simulink model "sliding_mode"  (R2025b)
settings: Solver=VariableStepAuto  StartTime=0.0  StopTime=50  RelTol=1e-3
libraries: simulink x2, slctrl_smc x1, matrix_library x1, cstblocks x1
settings Model: SimulationMode=rapid-accelerator  Creator=srivatsan  LastModifiedBy=srivatsan

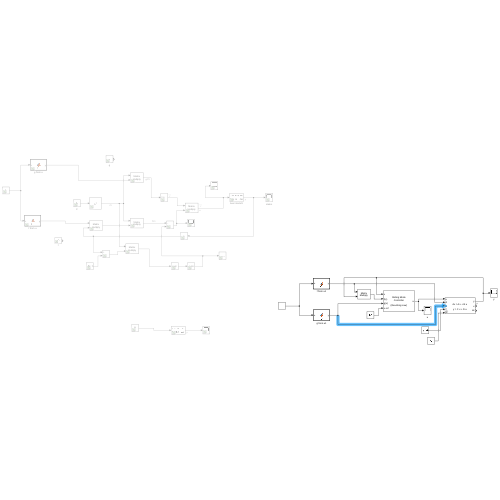
[thumbnail: Simulink's stored preview of the top-level diagram]
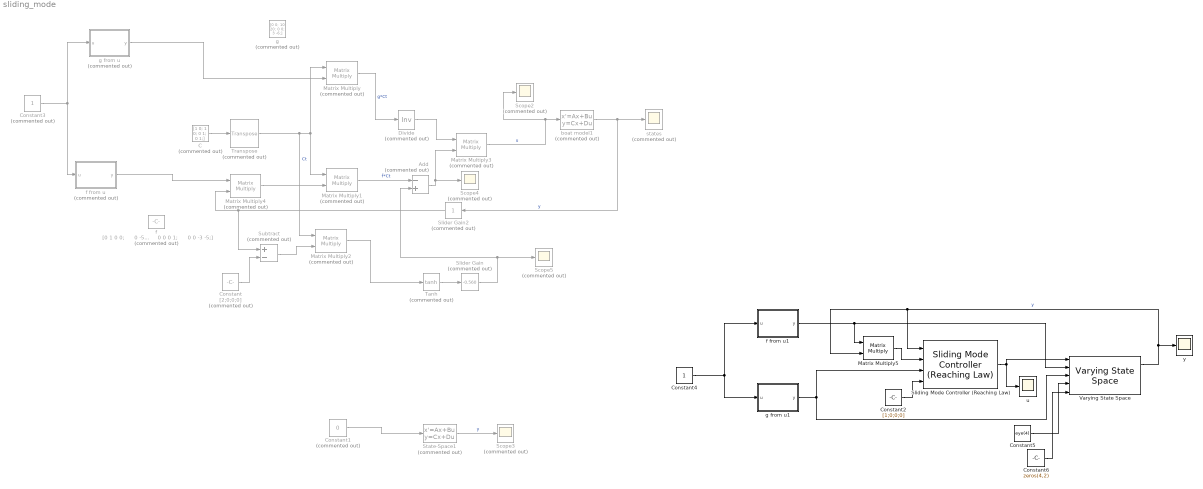
== system sliding_mode ==
  Add : Sum  Commented=on  Inputs=-+
  C : Constant  Commented=on  Value=[1 0; 1 0; 0 1; 0 1;]  VectorParams1D=off
  Constant : Constant  Commented=on  Value=[2;0;0;0]  VectorParams1D=off
  Constant1 : Constant  Commented=on  Value=0
  Constant2 : Constant  Value=[1;0;0;0]  VectorParams1D=off
  Constant3 : Constant  Commented=on
  Constant4 : Constant
  Constant5 : Constant  Value=eye(4)
  Constant6 : Constant  Value=zeros(4,2)
  Divide : Product  Commented=on  Inputs=/  Multiplication=Matrix(*)
  Matrix Multiply{,1..4} (5 alike) : Product  Commented=on  Multiplication=Matrix(*)
  Matrix Multiply5 : Product  Multiplication=Matrix(*)
  Scope{2..5} (4 alike) : Scope  Commented=on
      Scope2 settings: ActiveDisplayYMinimum=-0.20394139438387604  ActiveDisplayYMaximum=0.099478728460864418  DataLoggingVariableName=ScopeData2
      Scope3 settings: ActiveDisplayYMinimum=-7.1016769488332123  ActiveDisplayYMaximum=3.4136978035141685  DataLoggingVariableName=ScopeData3
      Scope4 settings: ActiveDisplayYMinimum=32.985672561237685  ActiveDisplayYMaximum=33.00453911435222  DataLoggingVariableName=ScopeData4
      Scope5 settings: ActiveDisplayYMinimum=-0.36552944112200225  ActiveDisplayYMaximum=0.6564815312712845  DataLoggingVariableName=ScopeData5
  Slider Gain : simulink/Math Operations/Slider Gain  Commented=on  gain=-0.560  low=-2  high=2
  Slider Gain2 : simulink/Math Operations/Slider Gain  Commented=on  gain=1  low=-2  high=2
  Sliding Mode Controller (Reaching Law) : slctrl_smc/Sliding Mode Controller (Reaching Law)  TaskMode=Tracking Mode  SlidingMatrix=[1 0;1 0;0 1;0 1]  EnableTrackingDerivative=off  EnableSwitchingFunction=off  ReachingLaw=Constant Rate  ReachingRate=1  ControlGain=0.01  PowerRate=0.01  BoundaryLayer=Hyperbolic Tangent  ZeroCross=off  Phi=0.01
  State-Space1 : StateSpace  Commented=on  A=[0,1;-10,-10]  B=[0;1;]  C=eye(2)  D=zeros(2,1)  InitialCondition=[5;3;]
  Subtract : Sum  Commented=on  Inputs=+-
  Tanh : Trigonometry  Commented=on  Operator=tanh
  Transpose : matrix_library/Transpose  Commented=on
  Varying State Space : cstblocks/Linear Parameter Varying/Varying State Space  InitialConditionSource=internal  InitialCondition=0  xNames=''  OutputX=on  OutputDX=on  Feedthrough=on  InputX0=off  InputDX0=off  InputU0=off  InputY0=off
  boat model1 : StateSpace  Commented=on  A=|  B=|  C=eye(4)  D=zeros(4,2)  InitialCondition=[0;0;1;0]
      A=|
      | [0 1 0 0;
      |      0 -5 30 0;
      |      0 0 0 1;
      |      0 0 -3 -5;]
      B=|
      | [0 0;
      |      10 20;
      |      0 0;
      |      3 -6;]
  f : Constant  Commented=on  Value=|
      | [0 1 0 0;
      |      0 -5 30 0;
      |      0 0 0 1;
      |      0 0 -3 -5;]
  f from u : MATLAB Function  Commented=on  TreatAsAtomicUnit=on
  f from u1 : MATLAB Function  TreatAsAtomicUnit=on
  g : Constant  Commented=on  Value=|  VectorParams1D=off
      | [0 0;
      |      10 20;
      |      0 0;
      |      3 -6;]
  g from u : MATLAB Function  Commented=on  TreatAsAtomicUnit=on
  g from u1 : MATLAB Function  TreatAsAtomicUnit=on
  states : Scope  Commented=on
      settings: ActiveDisplayYMinimum=-0.39772767591902924  ActiveDisplayYMaximum=2.2667310378705712
  u : Scope
      settings: ActiveDisplayYMinimum=-0.76850451056178137  ActiveDisplayYMaximum=0.49511973463973907  DataLoggingVariableName=ScopeData7
  y : Scope
      settings: ActiveDisplayYMinimum=-0.17359496071581337  ActiveDisplayYMaximum=1.1389480840558757  DataLoggingVariableName=ScopeData6
  wires:
  C/1 -> Transpose/1
  Transpose/1 -> Matrix Multiply2/1, Matrix Multiply/1, Matrix Multiply1/1  "Ct"
  boat model1/1 -> Slider Gain2/1, states/1  "y"
  Tanh/1 -> Slider Gain/1
  Matrix Multiply1/1 -> Add/1  "f*Ct"
  Divide/1 -> Matrix Multiply3/1
  Add/1 -> Matrix Multiply3/2, Scope4/1
  Matrix Multiply/1 -> Divide/1  "g*Ct"
  Matrix Multiply4/1 -> Matrix Multiply1/2
  Constant1/1 -> State-Space1/1
  State-Space1/1 -> Scope3/1  "y"
  Slider Gain/1 -> Add/2, Scope5/1
  Sliding Mode Controller (Reaching Law)/1 -> Varying State Space/1, u/1
  Matrix Multiply5/1 -> Sliding Mode Controller (Reaching Law)/2
  Constant2/1 -> Sliding Mode Controller (Reaching Law)/4
  Slider Gain2/1 -> Subtract/1, Matrix Multiply4/2
  Matrix Multiply2/1 -> Tanh/1
  Constant/1 -> Subtract/2
  Subtract/1 -> Matrix Multiply2/2
  Matrix Multiply3/1 -> Scope2/1, boat model1/1  "u"
  Constant3/1 -> g from u/1(u), f from u/1(u)
  f from u/1(y) -> Matrix Multiply4/1
  g from u/1(y) -> Matrix Multiply/2
  Constant4/1 -> f from u1/1(u), g from u1/1(u)
  f from u1/1(y) -> Varying State Space/2, Matrix Multiply5/1
  g from u1/1(y) -> Varying State Space/3, Sliding Mode Controller (Reaching Law)/3
  Varying State Space/1 -> Matrix Multiply5/2, Sliding Mode Controller (Reaching Law)/1, y/1  "y"
  Constant5/1 -> Varying State Space/4
  Constant6/1 -> Varying State Space/5

== matlab function sliding_mode/f from u ==
  data: u input; y output
function y = fcn(u)


y = [0 1 0 0;
     0 -5 30 0;
     0 0 0 1;
     0 0 -3 -5;];

== matlab function sliding_mode/f from u1 ==
  data: u input; y output
function y = fcn(u)


y = [0 1 0 0;
     0 -5 30 0;
     0 0 0 1;
     0 0 -3 -5;];

== matlab function sliding_mode/g from u1 ==
  data: u input; y output
function y = fcn(u)

m = 1;
I1 = 1;

d1 = 0.3;
d2 = 0.3;

L1 = 10;
L2 = 10;


y = [0 0;
     10 21;
     0 0;
     3 -6;];

== matlab function sliding_mode/g from u ==
  data: u input; y output
function y = fcn(u)

m = 1;
I1 = 1;

d1 = 0.3;
d2 = 0.3;

L1 = 10;
L2 = 10;


y = [0 0;
     10 20;
     0 0;
     3 -6;];
